simulink model "Total_Pjt"  (R2025b)
settings: Solver=FixedStepAuto  StartTime=0.0  StopTime=10.0  FixedStep=Ts  RelTol=1e-3
InitFcn:
  | para
values from neighbouring files (symbols this model uses):
  Ts = 0.01    [para.m]
settings Model: Creator=User  LastModifiedBy=User

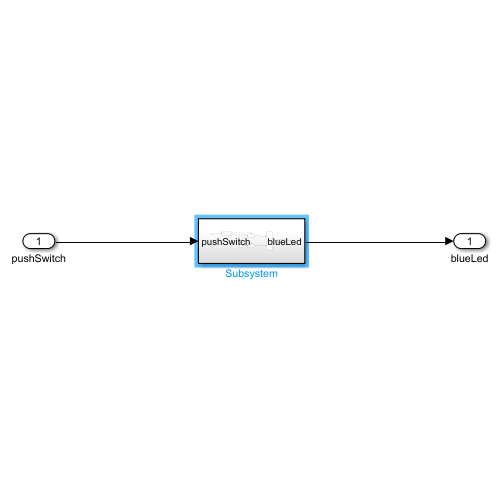
[thumbnail: Simulink's stored preview of the top-level diagram]
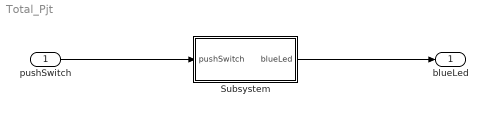
== system Total_Pjt ==
  pushSwitch : Inport  OutDataTypeStr=boolean
  Subsystem : Subsystem
  blueLed : Outport  OutMin=0  OutMax=50000  OutDataTypeStr=uint16
  wires:
  pushSwitch/1 -> Subsystem/1(pushSwitch)
  Subsystem/1(blueLed) -> blueLed/1

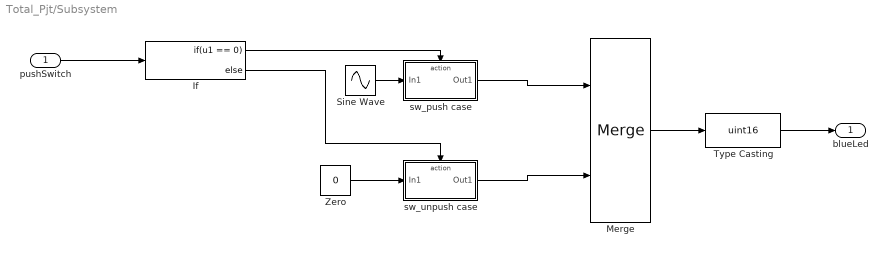
== system Total_Pjt/Subsystem ==
  pushSwitch : Inport
  If : If  IfExpression=u1 == 0
  Merge : Merge
  Sine Wave : Sin  SineType=Sample based  Amplitude=25000  Bias=25000  Samples=300  SampleTime=Ts
  Type Casting : DataTypeConversion  OutDataTypeStr=uint16  SaturateOnIntegerOverflow=off  RndMeth=Floor
  Zero : Constant  Value=0  OutDataTypeStr=Inherit: Inherit via back propagation
  sw_push case : Subsystem  TreatAsAtomicUnit=on
  sw_unpush case : Subsystem  TreatAsAtomicUnit=on
  blueLed : Outport  OutMax=50000
  wires:
  pushSwitch/1 -> If/1
  If/1 -> sw_push case/Action
  If/2 -> sw_unpush case/Action
  Zero/1 -> sw_unpush case/1(In1)
  Sine Wave/1 -> sw_push case/1(In1)
  sw_push case/1(Out1) -> Merge/1
  sw_unpush case/1(Out1) -> Merge/2
  Merge/1 -> Type Casting/1
  Type Casting/1 -> blueLed/1

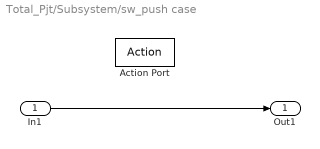
== system Total_Pjt/Subsystem/sw_push case ==
  In1 : Inport
  Action Port : ActionPort  ActionPortLabel=if(u1 == 0)
  Out1 : Outport
  wires:
  In1/1 -> Out1/1

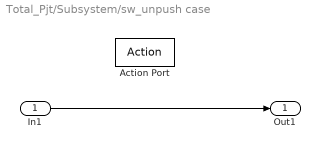
== system Total_Pjt/Subsystem/sw_unpush case ==
  In1 : Inport
  Action Port : ActionPort  ActionPortLabel=else
  Out1 : Outport
  wires:
  In1/1 -> Out1/1
